simulink model "PR_data"  (R2024a)
settings: Solver=ode45  StartTime=0.0  StopTime=stoptime  RelTol=1e-3
values from neighbouring files (symbols this model uses):
  amp_factor = [0.15; 0.03]/pi*180    [robotparam.m]
  I_est = 1e-3    (= 0.001)    [robotparam.m]
  ifreslosetrack = false    [robotparam.m]    (also in run_data_kick.m; run_data_losetrack.m = true; run_data_noise.m)
  ifresnoise = false    [robotparam.m]    (also in run_data_kick.m; run_data_losetrack.m; run_data_noise.m = true)
  ifrobotkicking = false    [robotparam.m]    (also in run_data_kick.m = true; run_data_losetrack.m; run_data_noise.m; run_sim.m = true)
  ifrobotnoise = false    [robotparam.m]    (also in run_data_kick.m; run_data_losetrack.m; run_data_noise.m = true)
  motor1mid = 0.445*180    (= 80.1)    [robotparam.m]    (also in run_receive.m)
  motor2mid = 0.45*180    (= 81)    [robotparam.m]    (also in run_receive.m)
  ref_theta = 0    [robotparam.m]    (also in run_data_kick.m = 3.14159265359; run_data_losetrack.m = 3.14159265359; run_data_noise.m = 3.14159265359; run_sim.m = 3.14159265359)
  ref_thetadot = 0    [robotparam.m]    (also in run_data_kick.m; run_data_losetrack.m; run_data_noise.m; run_sim.m)
  res_losetrack_period = 5    [robotparam.m]    (also in run_data_kick.m; run_data_losetrack.m = list(i,2); run_data_noise.m)
  res_losetrack_start = 9    [robotparam.m]    (also in run_data_kick.m; run_data_losetrack.m = list(i,1); run_data_noise.m)
  res_noise_seed = round(10000*[rand() rand()])    [robotparam.m]    (also in run_data_kick.m; run_data_losetrack.m; run_data_noise.m = [list(i,4) list(i,5)])
  res_noise_variance = 0.01*[1 1]    [robotparam.m]    (also in run_data_kick.m; run_data_losetrack.m; run_data_noise.m = [list(i,3) list(i,3)])
  robot_kick_height = 0    [robotparam.m]    (also in run_data_kick.m; run_data_losetrack.m; run_data_noise.m; run_sim.m = 1)
  robot_kick_period = 0.1    [robotparam.m]    (also in run_data_kick.m; run_data_losetrack.m; run_data_noise.m; run_sim.m)
  robot_kick_start = 10    [robotparam.m]    (also in run_data_kick.m = 30; run_data_losetrack.m; run_data_noise.m; run_sim.m = 1020)
  robot_noise_seed = round(10000*rand())    [robotparam.m]    (also in run_data_kick.m; run_data_losetrack.m; run_data_noise.m = list(i,2))
  robot_noise_variance = 0.0001    [robotparam.m]    (also in run_data_kick.m; run_data_losetrack.m; run_data_noise.m = list(i,1))
  robot_pendepth = 0.02    [robotparam.m]
  robot_penlength = 0.20    (= 0.2)    [robotparam.m]
  robot_penwidth = 0.02    [robotparam.m]
  robot_pulse_freq = 0.05    [robotparam.m]    (also in run_data_kick.m = list(i,1); run_data_losetrack.m = 0.5; run_data_noise.m = 0.5; run_sim.m = 0.01)
  robot_pulse_hight = 0.5    [robotparam.m]    (also in run_data_kick.m = list(i,2); run_data_losetrack.m; run_data_noise.m; run_sim.m = 0.08)
  robot_pulse_period = 0.1*100    (= 10)    [robotparam.m]    (also in run_data_kick.m; run_data_losetrack.m; run_data_noise.m; run_sim.m)
  robot_pulse_start = 60    [robotparam.m]    (also in run_data_kick.m = 30; run_data_losetrack.m = 10; run_data_noise.m = 10; run_sim.m = 1020)
  robot_sphere_mass = 0.1    [robotparam.m]
  s = {s1, s2}    [run_receive.m]
  samplingrate = 0.01    [robotparam.m]
  torquelim = 0.25*robot_penrho*robot_penlength*robot_penwidth*robot_pendepth*robot_penlength/2*g    (= 0.0196133)    [robotparam.m]
  Wout = 0*ones(3,1+4+2)    [robotparam.m]    (also in trainres.m = Woutmat)
  X = SS([1:3 6:end],:)    [trainres.m]
  Y = tar{i}    [trainres.m]
undefined symbols (not defined in the file or in its folder): arm_radius, arm_radius_previus, spring_position_scale, Z
libraries: sm_lib x9, nesl_utility x6, slrealtimeiplib x4, simulink x2, sldrtlib x1, slrealtimeutilitieslib x1, dspindex x1
settings Model: Creator=dante  LastModifiedBy=dante
settings SolverCC: AutoInsertRateTranBlk=on
settings OptimizationCC: DefaultParameterBehavior=Inlined  EnhancedBackFolding=on  PassReuseOutputArgsAs=Individual arguments  ZeroExternalMemoryAtStartup=off  ZeroInternalMemoryAtStartup=off  MaxStackSize=64  OptimizeBlockOrder=speed  DifferentSizesBufferReuse=on  OptimizationCustomize=off  EfficientTunableParamExpr=on
settings DebuggingCC: AlgebraicLoopMsg=none  ParameterTunabilityLossMsg=error
settings HardwareCC: ProdBitPerInt=16  ProdBitPerPointer=16  ProdBitPerSizeT=16  ProdBitPerPtrDiffT=16  ProdLargestAtomicFloat=None  ProdWordSize=8  ProdHWDeviceType=Atmel->AVR
settings SFSimCC: MATLABDynamicMemAlloc=off
settings RTWCC: Description=Embedded Coder  SystemTargetFile=ert.tlc  TemplateMakefile=ert_default_tmf  Toolchain=Arduino AVR  BuildConfiguration=Faster Runs
settings CodeAppCC: ForceParamTrailComments=on  IgnoreCustomStorageClasses=off  OperatorAnnotations=on  SimulinkDataObjDesc=on  SFDataObjDesc=on  InsertBlockDesc=on
settings ERTTargetCC: SupportContinuousTime=on  ExtModeTransport=3  ExtModeStaticAlloc=on  ExtModeStaticAllocSize=250  ExtModeMexFile=ext_xcp  ExtModeIntrfLevel=Level2 - Open  ERTCustomFileTemplate=example_file_process.tlc
settings ExplorerConfigSet: InternalSimMechanicsExplorerSettings="<ExplorerConfiguration><canonicalview>default</canonicalview><AnimationSetting><BasePlaybackSpeed>1.0</BasePlaybackSpeed><PlaybackSpeedFactor>1.0</PlaybackSpeedFactor></AnimationSetting><TilePanel><TileInfo><Tiles Columns=\"1\" Count=\"1\" Rows=\"1\"><Column Weight=\"1\"/><Row Weight=\"1\"/><Tile Height=\"1\" Width=\"1\" X=\"0\" Y=\"0\"/></Tiles></TileInfo><SceneInfo><SceneViewer><BGColor><R>1</R><G>1</G><B>1</B></BGColor><Camera><DoPerspective>off</DoPerspective><Position><X>-6.72546141640504441e-05</X><Y>-1.00004999683291818</Y><Z>0.290146129229805205</Z></Position><Center><X>-6.72546141640504441e-05</X><Y>-4.99968329182032267e-05</Y><Z>0.290146129229805205</Z></Center><Up><X>0</X><Y>-0</Y><Z>1</Z></Up><ViewLimDist>1</ViewLimDist><YLim>0.252627686260521567</YLim><XLim>0.252627686260521567</XLim></Camera></SceneViewer></SceneInfo></TilePanel><MechEditorPanel><Cameras/><GfxPanelCameraMap/><VideoCreator><PlaybackSpeedRatio>1.0</PlaybackSpeedRatio><FrameRate>30</FrameRate><VideoFormat>Motion JPEG AVI</VideoFormat><FrameSize>auto</FrameSize></VideoCreator></MechEditorPanel></ExplorerConfiguration>"

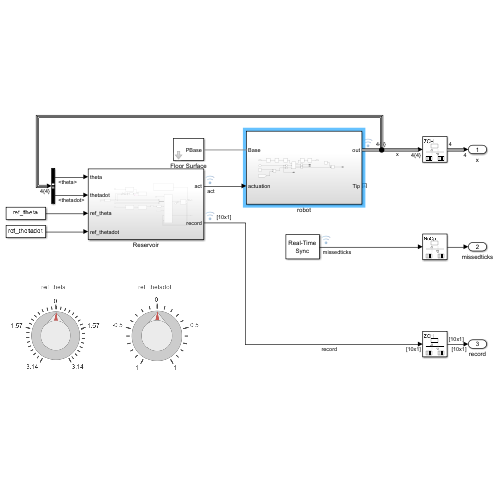
[thumbnail: Simulink's stored preview of the top-level diagram]
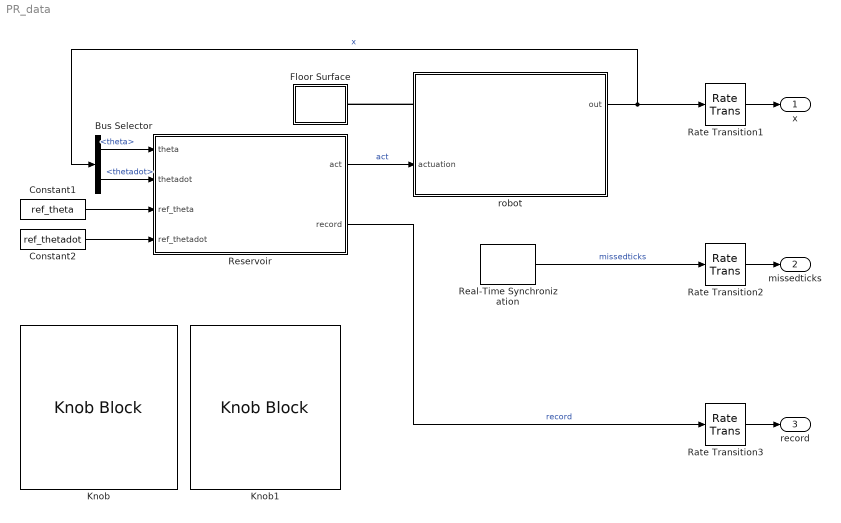
== system PR_data ==
  Bus Selector : BusSelector  OutputSignals=theta,thetadot
  Constant1 : Constant  Value=ref_theta
  Constant2 : Constant  Value=ref_thetadot
  Floor Surface : Subsystem  mask{length=0.5, width=0.5}
      mask prompts: length "grid length [m]"; width "grid width [m]"
  Knob : KnobBlock  ScaleMin=-3.14  ScaleMax=3.14  TickInterval=1.57
  Knob1 : KnobBlock  ScaleMin=-1  ScaleMax=1  TickInterval=0.5
  Rate Transition1 : RateTransition  OutPortSampleTime=samplingrate
  Rate Transition2 : RateTransition  OutPortSampleTime=samplingrate
  Rate Transition3 : RateTransition  OutPortSampleTime=samplingrate
  Real-Time Synchronization : sldrtlib/Real-Time Synchronization  SampleTime=samplingrate  MaxMissedTicks=1000  ShowMissedTicks=on  YieldWhenWaiting=off
  Reservoir : Subsystem
  robot : Subsystem
      settings: PortSchema="{\"entries\":[{\"content\":{\"sides\":[{\"content\":{\"connectorIds\":[\"LConn1\",\"In1\"]},\"type\":\"ConnectorPlacement.EquallySpacedRectSide\",\"uuid\":\"dab85734-5223-47c8-98b4-c5bd2646397a\"},{\"content\":{\"connectorIds\":[\"Out1\",\"RConn1\"],\"side\":\"RIGHT\"},\"type\":\"ConnectorPlacement.EquallySpacedRectSide\",\"uuid\":\"c0ea15e2-5ad4-47fa-8aeb-0218d5c494db\"},{\"content\":{\"side\":\"TOP\"},\"type\":\"ConnectorPlacement.EquallySpacedRectSide\",\"uuid\":\"166100d5-86a1-4512-901d-80935eea9023\"}]},\"type\":\"ConnectorPlacement.EquallySpacedConnector\",\"uuid\":\"1b956e2c-5409-4c92-995b-8a7c87877ed0\"}],\"packageUris\":[\"http://schema.mathworks.com/mf0/Connector/R2020b\"],\"version\":\"1.0\"}"
  x : Outport
  missedticks : Outport  Port=2
  record : Outport  Port=3
  wires:
  robot/1(out) -> Bus Selector/1, Rate Transition1/1  "x"
  Real-Time Synchronization/1 -> Rate Transition2/1  "missedticks"
  Constant2/1 -> Reservoir/4(ref_thetadot)
  Constant1/1 -> Reservoir/3(ref_theta)
  Reservoir/2(record) -> Rate Transition3/1  "record"
  Rate Transition1/1 -> x/1
  Rate Transition2/1 -> missedticks/1
  Rate Transition3/1 -> record/1
  Bus Selector/1 -> Reservoir/1(theta)  "<theta>"
  Bus Selector/2 -> Reservoir/2(thetadot)  "<thetadot>"
  Reservoir/1(act) -> robot/1(actuation)  "act"
  connections:
  robot/LConn1 -- Floor Surface/RConn1

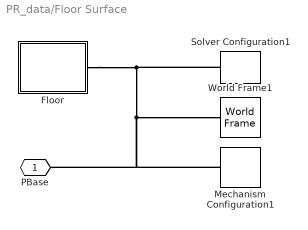
== system PR_data/Floor Surface ==
  Floor : Subsystem
  Mechanism Configuration1 : sm_lib/Utilities/Mechanism Configuration  UniformGravity=Constant  GravityVector=[0 0 -9.80665]  GravityVectorUnits=m/s^2  LinearizationDelta=0.001  JointModeTransitionNonlinearIterations=2
  Solver Configuration1 : nesl_utility/Solver Configuration  PhysicalDomain=network_engine_domain  SubClassName=solver  LeftPortType=input  RightPortType=generic  Tones=[]  Harmonics=[]  SimulateNoise=off  Profile=off  UseLocalSampling=off  EnableSwitchedLinearOptims=on  FrequencyDomain=off  UseCCode=off  RelTol=0.001  AbsTol=1e-06  MinStep=1e-09  ToWorkspace=off  RevertToSquareIcSolve=off  NumHomotopyIterations=100  PhasorMode=off  PhasorModeNumHarmonics=1  ConsistencySolver=NEWTON_FTOL  IndexReductionMethod=DerivativeReplacement  DoDC=off  ResidualTolerance=1e-09  ConsistencyTolSource=GLOBAL  ConsistencyAbsTol=0.001  ConsistencyRelTol=0.001  ConsistencyTolFactor=0.001  UseLocalSolver=off  LocalSolverChoice=NE_BACKWARD_EULER_ADVANCER  ResolveIndetEquations=on  FunctionEvalNumThread=1  LocalSolverSampleTime=0.0002  DoFixedCost=off  MaxNonlinIter=10  MaxModeIter=2  ComputeImpulses=off  ImpulseIterations=2  LinearAlgebra=Sparse  LinearAlgebraNumThread=0  EquationFormulation=NE_TIME_EF  DelaysMemoryBudget=1024  AutomaticFiltering=off  FilteringTimeConstant=0.001  PartitionStorageMethod=AS_NEEDED  PartitionMemoryBudget=1024  PartitionMethod=FAST  MultibodyUseLocalSolver=off  MultibodyLocalSolverChoice=ODE1  MultibodyLocalSolverSampleTime=0.001
  World Frame1 : sm_lib/Frames and Transforms/World Frame
  PBase : PMIOPort  Side=Right
  connections:
  Floor/RConn1 -- PBase/RConn1 -- Mechanism Configuration1/RConn1 -- World Frame1/RConn1 -- Solver Configuration1/RConn1

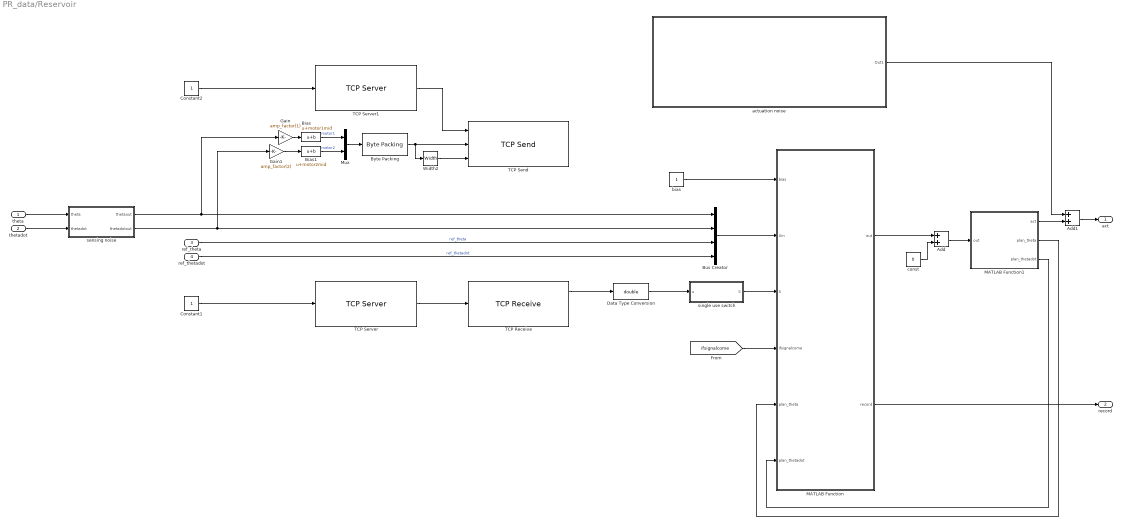
== system PR_data/Reservoir ==
  theta : Inport
  thetadot : Inport  Port=2
  ref_theta : Inport  Port=3
  ref_thetadot : Inport  Port=4
  Add : Sum
  Add1 : Sum
  Bias : Bias  Bias=motor1mid  SaturateOnIntegerOverflow=off
  Bias1 : Bias  Bias=motor2mid  SaturateOnIntegerOverflow=off
  Bus Creator : BusCreator  Inputs=4
  "Byte Packing " : slrealtimeutilitieslib/Byte Packing  MaskPackedDataType=uint8  MaskUnpackedDataTypes={'double'}  MaskAlignment=1
  Constant1 : Constant
  Constant2 : Constant
  Data Type Conversion : DataTypeConversion  OutDataTypeStr=double  SaturateOnIntegerOverflow=off  RndMeth=Floor
  Gain : Gain  Gain=amp_factor(1)
  Gain1 : Gain  Gain=amp_factor(2)
  MATLAB Function : MATLAB Function  TreatAsAtomicUnit=on
  MATLAB Function1 : MATLAB Function  TreatAsAtomicUnit=on
  Mux : Mux  Inputs=2
  TCP Receive : slrealtimeiplib/TCP Receive  socketAddPortVal=Server: 169.254.170.51:65432  rcvWidth=2  sampleTime=-1
  TCP Send : slrealtimeiplib/TCP Send  socketAddPortVal=Server: 169.254.170.51:65431  sampleTime=-1
  TCP Server : slrealtimeiplib/TCP Server  Priority=-1  useHostTargetConn=off  serverAddress=169.254.170.51  serverPort=65432
  TCP Server1 : slrealtimeiplib/TCP Server  Priority=-1  useHostTargetConn=off  serverAddress=169.254.170.51  serverPort=65431
  Width2 : Width
  actuation noise : Subsystem
  bias : Constant
  const : Constant  Value=0
  sensing noise : Subsystem
  single use switch : Subsystem
  act : Outport
  record : Outport  Port=2
  wires:
  TCP Server/1 -> TCP Receive/1
  Constant1/1 -> TCP Server/1
  ref_thetadot/1 -> Bus Creator/4  "ref_thetadot"
  ref_theta/1 -> Bus Creator/3  "ref_theta"
  Bus Creator/1 -> MATLAB Function/2(Xin)
  TCP Receive/1 -> Data Type Conversion/1
  bias/1 -> MATLAB Function/1(bias)
  MATLAB Function/1(out) -> Add/1
  const/1 -> Add/2
  Add/1 -> MATLAB Function1/1(out)
  MATLAB Function/2(record) -> record/1
  Mux/1 -> "Byte Packing "/1
  Width2/1 -> TCP Send/3
  "Byte Packing "/1 -> Width2/1, TCP Send/2
  Gain/1 -> Bias/1
  Gain1/1 -> Bias1/1
  Bias1/1 -> Mux/2  "motor2"
  Bias/1 -> Mux/1  "motor1"
  Constant2/1 -> TCP Server1/1
  TCP Server1/1 -> TCP Send/1
  Data Type Conversion/1 -> single use switch/1(u)
  single use switch/1(S) -> MATLAB Function/3(S)
  MATLAB Function1/2(plan_theta) -> MATLAB Function/5(plan_theta)
  MATLAB Function1/3(plan_thetadot) -> MATLAB Function/6(plan_thetadot)
  [ifsignalcome] -> MATLAB Function/4(ifsignalcome)
  MATLAB Function1/1(act) -> Add1/2
  Add1/1 -> act/1
  actuation noise/1(Out1) -> Add1/1
  sensing noise/1(thetaout) -> Bus Creator/1, Gain/1
  sensing noise/2(thetadotout) -> Bus Creator/2, Gain1/1
  theta/1 -> sensing noise/1(theta)
  thetadot/1 -> sensing noise/2(thetadot)

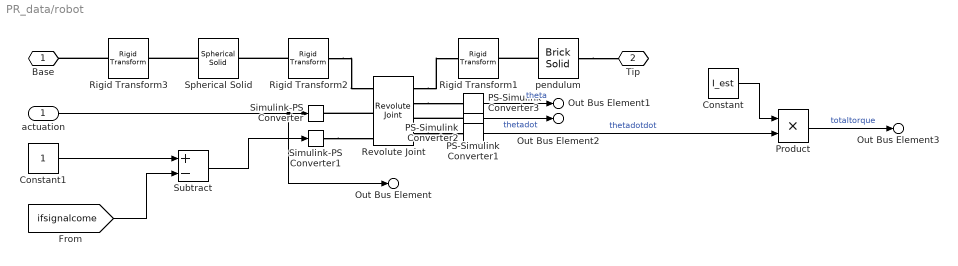
== system PR_data/robot ==
  actuation : Inport
  Constant : Constant  Value=I_est
  Constant1 : Constant
  PS-Simulink Converter1 : nesl_utility/PS-Simulink Converter  PhysicalDomain=network_engine_domain  SubClassName=ps_output  LeftPortType=input  RightPortType=output  PseudoPeriodic=off  Frequencies=[]  VectorFormat=1-D array  Unit=1  AffineConversion=off
  PS-Simulink Converter2 : nesl_utility/PS-Simulink Converter  PhysicalDomain=network_engine_domain  SubClassName=ps_output  LeftPortType=input  RightPortType=output  PseudoPeriodic=off  Frequencies=[]  VectorFormat=1-D array  Unit=1  AffineConversion=off
  PS-Simulink Converter3 : nesl_utility/PS-Simulink Converter  PhysicalDomain=network_engine_domain  SubClassName=ps_output  LeftPortType=input  RightPortType=output  PseudoPeriodic=off  Frequencies=[]  VectorFormat=1-D array  Unit=1  AffineConversion=off
  Product : Product
  Revolute Joint : sm_lib/Joints/Revolute Joint  JointMode=ProvidedByInput  CompositeWrenchDir=FollowerOnBase  CompositeWrenchFrame=BaseFrame  SenseConstraintForce=off  SenseConstraintTorque=off  SenseTotalForce=off  SenseTotalTorque=off  PositionTargetSpecify=on  PositionTargetPriority=Low  PositionTargetValue=robot_ini_theta_p  PositionTargetValueUnits=rad  VelocityTargetSpecify=on  VelocityTargetPriority=Low  VelocityTargetValue=robot_ini_thetadot_p  VelocityTargetValueUnits=rad/s  EquilibriumPosition=0  EquilibriumPositionUnits=rad  SpringStiffness=0  SpringStiffnessUnits=N*m/rad  DampingCoefficient=robot_damping_coeff  DampingCoefficientUnits=N*m/(rad/s)  LowerLimitSpecify=off  LowerLimitBound=-90  LowerLimitBoundUnits=deg  LowerLimitStiffness=1e4  LowerLimitStiffnessUnits=N*m/deg  LowerLimitDamping=10  LowerLimitDampingUnits=N*m/(deg/s)  LowerLimitTransitionRegionWidth=0.1  LowerLimitTransitionRegionWidthUnits=deg  UpperLimitSpecify=off  UpperLimitBound=90  UpperLimitBoundUnits=deg  UpperLimitStiffness=1e4  UpperLimitStiffnessUnits=N*m/deg  UpperLimitDamping=10  UpperLimitDampingUnits=N*m/(deg/s)  UpperLimitTransitionRegionWidth=0.1  UpperLimitTransitionRegionWidthUnits=deg  TorqueActuationMode=InputTorque  MotionActuationMode=ComputedMotion  SensePosition=on  SenseVelocity=on  SenseAcceleration=on  SenseTorqueForce=off  SenseLowerLimitTorqueForce=off  SenseUpperLimitTorqueForce=off
  Rigid Transform1 : sm_lib/Frames and Transforms/Rigid Transform  RotationMethod=AlignedAxes  FollAlignAxisA=+X  BaseAlignAxisA=+X  FollAlignAxisB=-Z  BaseAlignAxisB=+Y  RotationStandardAxis=+Z  RotationAngle=180  RotationAngleUnits=deg  RotationArbitraryAxis=[0 0 1]  RotationSequenceAxes=FollowerAxes  RotationSequence=XYX  RotationSequenceAngles=[0 0 0]  RotationSequenceAnglesUnits=deg  RotationMatrix=[1 0 0; 0 1 0; 0 0 1]  Quaternion=[1 0 0 0]  TranslationMethod=None  TranslationCartesianOffset=[arm_radius*spring_position_scale 0 0]  TranslationCartesianOffsetUnits=m  TranslationStandardAxis=+Z  TranslationStandardOffset=0  TranslationStandardOffsetUnits=m  TranslationROffset=arm_radius_previus*spring_position_scale  TranslationROffsetUnits=m  TranslationThetaOffset=theta  TranslationThetaOffsetUnits=deg  TranslationZOffset=0  TranslationZOffsetUnits=m
  Rigid Transform2 : sm_lib/Frames and Transforms/Rigid Transform  RotationMethod=AlignedAxes  FollAlignAxisA=+X  BaseAlignAxisA=+X  FollAlignAxisB=+Y  BaseAlignAxisB=+Z  RotationStandardAxis=+Z  RotationAngle=180  RotationAngleUnits=deg  RotationArbitraryAxis=[0 0 1]  RotationSequenceAxes=FollowerAxes  RotationSequence=XYX  RotationSequenceAngles=[0 0 0]  RotationSequenceAnglesUnits=deg  RotationMatrix=[1 0 0; 0 1 0; 0 0 1]  Quaternion=[1 0 0 0]  TranslationMethod=None  TranslationCartesianOffset=[arm_radius*spring_position_scale 0 0]  TranslationCartesianOffsetUnits=m  TranslationStandardAxis=+Z  TranslationStandardOffset=0  TranslationStandardOffsetUnits=m  TranslationROffset=arm_radius_previus*spring_position_scale  TranslationROffsetUnits=m  TranslationThetaOffset=theta  TranslationThetaOffsetUnits=deg  TranslationZOffset=0  TranslationZOffsetUnits=m
  Rigid Transform3 : sm_lib/Frames and Transforms/Rigid Transform  RotationMethod=None  FollAlignAxisA=+X  BaseAlignAxisA=+X  FollAlignAxisB=+Y  BaseAlignAxisB=+Z  RotationStandardAxis=+Z  RotationAngle=180  RotationAngleUnits=deg  RotationArbitraryAxis=[0 0 1]  RotationSequenceAxes=FollowerAxes  RotationSequence=XYX  RotationSequenceAngles=[0 0 0]  RotationSequenceAnglesUnits=deg  RotationMatrix=[1 0 0; 0 1 0; 0 0 1]  Quaternion=[1 0 0 0]  TranslationMethod=StandardAxis  TranslationCartesianOffset=[arm_radius*spring_position_scale 0 0]  TranslationCartesianOffsetUnits=m  TranslationStandardAxis=+Z  TranslationStandardOffset=robot_penposz  TranslationStandardOffsetUnits=m  TranslationROffset=arm_radius_previus*spring_position_scale  TranslationROffsetUnits=m  TranslationThetaOffset=theta  TranslationThetaOffsetUnits=deg  TranslationZOffset=0  TranslationZOffsetUnits=m
  Simulink-PS Converter : nesl_utility/Simulink-PS Converter  PhysicalDomain=network_engine_domain  SubClassName=ps_input  LeftPortType=input  RightPortType=output  PseudoPeriodic=off  Frequencies=[]  NoiseDistribution=none  NoiseParameters=[]  Unit=1  AffineConversion=off  FilteringAndDerivatives=provide  SimscapeFilterOrder=1  InputFilterTimeConstant=0.001  UdotUserProvided=0
  Simulink-PS Converter1 : nesl_utility/Simulink-PS Converter  PhysicalDomain=network_engine_domain  SubClassName=ps_input  LeftPortType=input  RightPortType=output  PseudoPeriodic=off  Frequencies=[]  NoiseDistribution=none  NoiseParameters=[]  Unit=1  AffineConversion=off  FilteringAndDerivatives=zero  SimscapeFilterOrder=1  InputFilterTimeConstant=0.001  UdotUserProvided=0
  Spherical Solid : sm_lib/Body Elements/Spherical Solid  SphereRadius=robot_sphere_radius  SphereRadiusUnits=m  ExportEntireGeometry=off  InertiaType=CalculateFromGeometry  BasedOnType=Mass  Density=1000  DensityUnits=kg/m^3  Mass=robot_sphere_mass  MassUnits=kg  CenterOfMass=[0 0 0]  CenterOfMassUnits=m  MomentsOfInertia=[1 1 1]  MomentsOfInertiaUnits=kg*m^2  ProductsOfInertia=[0 0 0]  ProductsOfInertiaUnits=kg*m^2  GraphicType=FromGeometry  MarkerShape=Sphere  MarkerSize=10  GraphicVisPropType=SimpleVisualProperties  GraphicDiffuseColor=[0.8 0.8 0.8]  GraphicOpacity=1.0  GraphicSpecularColor=[0.5 0.5 0.5 1.0]  GraphicAmbientColor=[0.15 0.15 0.15 1.0]  GraphicEmissiveColor=[0.0 0.0 0.0 1.0]  GraphicShininess=75  DoExposeReferenceFrame=on  SerializedFrames=<Frames><Frame><Id>Frame1</Id><Value><Name>F1</Name><Origin><Source>ReferenceFrame</Source><FeatureName></FeatureName></Origin><PrimaryAxis><DefinedDirection>+Z</DefinedDirection><Source>ReferenceFrame</Source><SourceDirection>+Z</SourceDirection><FeatureName></FeatureName></PrimaryAxis><SecondaryAxis><DefinedDirection>+X</DefinedDirection><Source>ReferenceFrame</Source><SourceDirection>+X</SourceDirection><FeatureName></FeatureName></SecondaryAxis></Value></Frame></Frames>
  Subtract : Sum  Inputs=+-
  pendulum : sm_lib/Body Elements/Brick Solid  BrickDimensions=[robot_penwidth robot_pendepth robot_penlength]  BrickDimensionsUnits=m  ExportEntireGeometry=off  InertiaType=CalculateFromGeometry  BasedOnType=Density  Density=robot_penrho  DensityUnits=kg/m^3  Mass=1  MassUnits=kg  CenterOfMass=[0 0 0]  CenterOfMassUnits=m  MomentsOfInertia=[1 1 1]  MomentsOfInertiaUnits=kg*m^2  ProductsOfInertia=[0 0 0]  ProductsOfInertiaUnits=kg*m^2  GraphicType=FromGeometry  MarkerShape=Sphere  MarkerSize=10  GraphicVisPropType=SimpleVisualProperties  GraphicDiffuseColor=[0.0 0.4 1.0]  GraphicOpacity=1.0  GraphicSpecularColor=[0.5 0.5 0.5 1.0]  GraphicAmbientColor=[0.15 0.15 0.15 1.0]  GraphicEmissiveColor=[0.0 0.0 0.0 1.0]  GraphicShininess=75  DoExposeReferenceFrame=off  SerializedFrames=<Frames><Frame><Id>Frame1</Id><Value><Name>F1</Name><Origin><Source>GeometricFeature</Source><FeatureName>-z surface</FeatureName></Origin><PrimaryAxis><DefinedDirection>+Z</DefinedDirection><Source>ReferenceFrame</Source><SourceDirection>+Z</SourceDirection><FeatureName></FeatureName></PrimaryAxis><SecondaryAxis><DefinedDirection>+X</DefinedDirection><Source>ReferenceFrame</Source><SourceDirection>+X</SourceDirection><FeatureName></FeatureName></SecondaryAxis></Value></Frame><Frame><Id>Frame2</Id><Value><Name>F2</Name><Origin><Source>GeometricFeature</Source><FeatureName>+z surface</FeatureName></Origin><PrimaryAxis><DefinedDirection>+Z</DefinedDirection><Source>ReferenceFrame</Source><SourceDirection>-Z</SourceDirection><FeatureName></FeatureName></PrimaryAxis><SecondaryAxis><DefinedDirection>+X</DefinedDirection><Source>ReferenceFrame</Source><SourceDirection>+X</SourceDirection><FeatureName></FeatureName></SecondaryAxis></Value></Frame></Frames>
  Base : PMIOPort  Side=Left
  Tip : PMIOPort  Port=2  Side=Right
  Out Bus Element1 : Outport  PortName=out  Element=theta
  Out Bus Element2 : Outport  PortName=out  Element=thetadot
  Out Bus Element3 : Outport  PortName=out  Element=totaltorque
  Out Bus Element : Outport  PortName=out  Element=actuationtorque
  wires:
  PS-Simulink Converter3/1 -> Out Bus Element1/1  "theta"
  PS-Simulink Converter1/1 -> Out Bus Element2/1  "thetadot"
  PS-Simulink Converter2/1 -> Product/2  "thetadotdot"
  Product/1 -> Out Bus Element3/1  "totaltorque"
  Constant/1 -> Product/1
  actuation/1 -> Simulink-PS Converter/1, Out Bus Element/1
  Subtract/1 -> Simulink-PS Converter1/1
  Constant1/1 -> Subtract/1
  [ifsignalcome] -> Subtract/2
  connections:
  Revolute Joint/LConn2 -- Simulink-PS Converter/RConn1
  Revolute Joint/RConn2 -- PS-Simulink Converter3/LConn1
  Rigid Transform2/LConn1 -- Spherical Solid/RConn1
  PS-Simulink Converter1/LConn1 -- Revolute Joint/RConn3
  Spherical Solid/LConn1 -- Rigid Transform3/RConn1
  pendulum/LConn1 -- Rigid Transform1/RConn1
  Rigid Transform3/LConn1 -- Base/RConn1
  pendulum/RConn1 -- Tip/RConn1
  Rigid Transform2/RConn1 -- Revolute Joint/LConn1
  Revolute Joint/RConn4 -- PS-Simulink Converter2/LConn1
  Revolute Joint/RConn1 -- Rigid Transform1/LConn1
  Simulink-PS Converter1/RConn1 -- Revolute Joint/LConn3

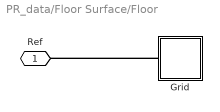
== system PR_data/Floor Surface/Floor ==
  Grid : Subsystem  mask(Grid Lines){grid_origin=[-length -width 0], grid_size=[length width], grid_linewidth=0.001, grid_num_squares=20, grid_color=[0.8 0.8 0.8], grid_opacity=0.8}
      mask prompts: grid_origin "Origin (m)"; grid_size "Arena size (m)"; grid_linewidth "Grid Line Width (m)"; grid_num_squares "Number of Squares"; grid_color "Grid Color [RGB]"; grid_opacity "Grid Opacity (0-1)"
      mask help: Creates grids on 3 planes XZ, YZ, and XZ.
      mask init:
      | mesh_xsec = Extr_Data_Mesh(grid_size(1), grid_size(2), grid_num_squares, grid_num_squares, grid_size(1)/grid_num_squares-grid_linewidth, grid_size(2)/grid_num_squares-grid_linewidth);
  Ref : PMIOPort  Side=Right
  connections:
  Grid/LConn1 -- Ref/RConn1

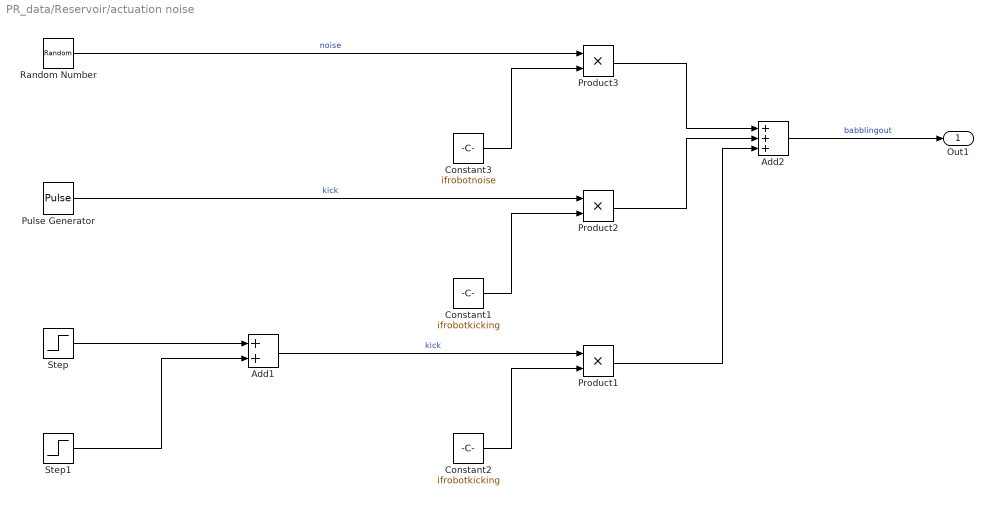
== system PR_data/Reservoir/actuation noise ==
  Add1 : Sum
  Add2 : Sum  Inputs=+++
  Constant1 : Constant  Value=ifrobotkicking
  Constant2 : Constant  Value=ifrobotkicking
  Constant3 : Constant  Value=ifrobotnoise
  Product1 : Product
  Product2 : Product
  Product3 : Product
  Pulse Generator : DiscretePulseGenerator  PulseType=Time based  Amplitude=robot_pulse_hight  Period=1/robot_pulse_freq  PulseWidth=robot_pulse_period*robot_pulse_freq  PhaseDelay=robot_pulse_start
  Random Number : RandomNumber  Variance=robot_noise_variance  Seed=robot_noise_seed  SampleTime=samplingrate
  Step : Step  Time=robot_kick_start  After=robot_kick_height  SampleTime=0
  Step1 : Step  Time=robot_kick_start+robot_kick_period  After=-robot_kick_height  SampleTime=0
  Out1 : Outport
  wires:
  Constant2/1 -> Product1/2
  Random Number/1 -> Product3/1  "noise"
  Product1/1 -> Add2/3
  Step/1 -> Add1/1
  Product2/1 -> Add2/2
  Product3/1 -> Add2/1
  Step1/1 -> Add1/2
  Pulse Generator/1 -> Product2/1  "kick"
  Add2/1 -> Out1/1  "babblingout"
  Constant1/1 -> Product2/2
  Constant3/1 -> Product3/2
  Add1/1 -> Product1/1  "kick"

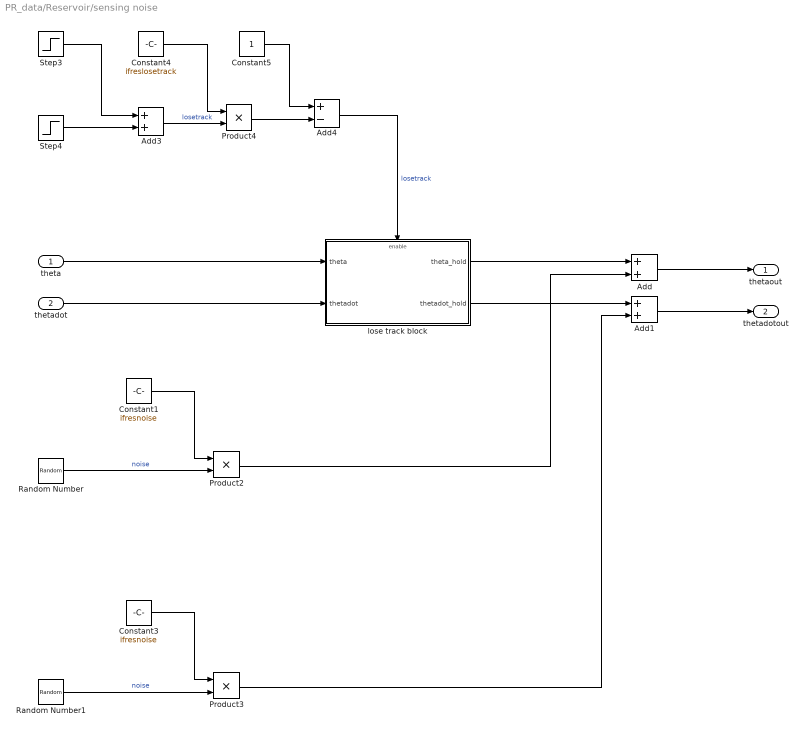
== system PR_data/Reservoir/sensing noise ==
  theta : Inport
  thetadot : Inport  Port=2
  Add : Sum
  Add1 : Sum
  Add3 : Sum
  Add4 : Sum  Inputs=+-
  Constant1 : Constant  Value=ifresnoise
  Constant3 : Constant  Value=ifresnoise
  Constant4 : Constant  Value=ifreslosetrack
  Constant5 : Constant
  Product2 : Product
  Product3 : Product
  Product4 : Product
  Random Number : RandomNumber  Variance=res_noise_variance(1)  Seed=res_noise_seed(1)  SampleTime=samplingrate
  Random Number1 : RandomNumber  Variance=res_noise_variance(2)  Seed=res_noise_seed(2)  SampleTime=samplingrate
  Step3 : Step  Time=res_losetrack_start  SampleTime=0
  Step4 : Step  Time=res_losetrack_start+res_losetrack_period  After=-1  SampleTime=0
  lose track block : Subsystem
  thetaout : Outport
  thetadotout : Outport  Port=2
  wires:
  Step3/1 -> Add3/1
  Add4/1 -> lose track block/Enable  "losetrack"
  Constant5/1 -> Add4/1
  Constant4/1 -> Product4/1
  Step4/1 -> Add3/2
  Product4/1 -> Add4/2
  Add3/1 -> Product4/2  "losetrack"
  thetadot/1 -> lose track block/2(thetadot)
  theta/1 -> lose track block/1(theta)
  Random Number1/1 -> Product3/2  "noise"
  Constant3/1 -> Product3/1
  Product3/1 -> Add1/2
  Constant1/1 -> Product2/1
  Random Number/1 -> Product2/2  "noise"
  Product2/1 -> Add/2
  lose track block/1(theta_hold) -> Add/1
  lose track block/2(thetadot_hold) -> Add1/1
  Add/1 -> thetaout/1
  Add1/1 -> thetadotout/1

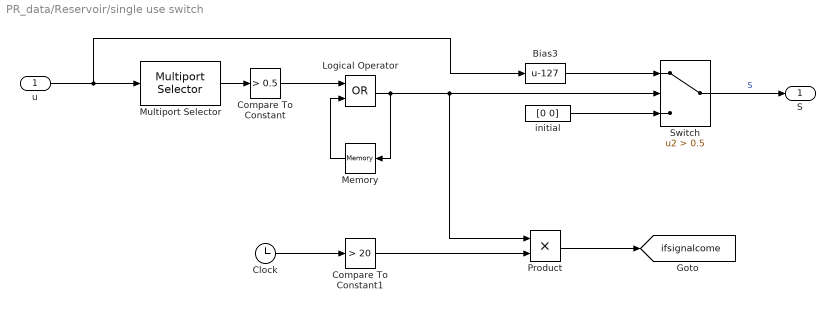
== system PR_data/Reservoir/single use switch ==
  u : Inport
  Bias3 : Bias  Bias=-127  SaturateOnIntegerOverflow=off
  Clock : Clock
  Compare To Constant : simulink/Logic and Bit Operations/Compare To Constant  relop=>  const=0.5  OutDataTypeStr=boolean
  Compare To Constant1 : simulink/Logic and Bit Operations/Compare To Constant  relop=>  const=20  OutDataTypeStr=boolean
  Logical Operator : Logic  Operator=OR  AllPortsSameDT=off  OutDataTypeStr=boolean
  Memory : Memory
  Multiport Selector : dspindex/Multiport Selector  rowsOrCols=Rows  idxCellArray=1  idxErrMode=Clip Index
  Product : Product
  Switch : Switch  Criteria=u2 > Threshold  Threshold=0.5  SaturateOnIntegerOverflow=off  InputSameDT=off
  initial : Constant  Value=[0 0]
  S : Outport
  tag scope: ifsignalcome=global
  wires:
  Switch/1 -> S/1  "S"
  Memory/1 -> Logical Operator/2
  initial/1 -> Switch/3
  Compare To Constant/1 -> Logical Operator/1
  Bias3/1 -> Switch/1
  u/1 -> Multiport Selector/1, Bias3/1
  Logical Operator/1 -> Switch/2, Product/1, Memory/1
  Multiport Selector/1 -> Compare To Constant/1
  Clock/1 -> Compare To Constant1/1
  Compare To Constant1/1 -> Product/2
  Product/1 -> [ifsignalcome]

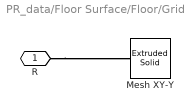
== system PR_data/Floor Surface/Floor/Grid ==
  Mesh XY-Y : sm_lib/Body Elements/Extruded Solid  ExtrusionType=General  PolygonNumSides=3  PolygonOuterRadius=1  PolygonOuterRadiusUnits=m  ExportEntireGeometry=off  ExtrusionCrossSection=mesh_xsec  ExtrusionCrossSectionUnits=m  ExportConvexHullGeometry=off  ExtrusionLength=grid_linewidth  ExtrusionLengthUnits=m  InertiaType=CalculateFromGeometry  BasedOnType=Density  Density=1000  DensityUnits=kg/(m^3)  Mass=1  MassUnits=kg  CenterOfMass=[0 0 0]  CenterOfMassUnits=m  MomentsOfInertia=[1 1 1]  MomentsOfInertiaUnits=kg*m^2  ProductsOfInertia=[0 0 0]  ProductsOfInertiaUnits=kg*m^2  GraphicType=FromGeometry  MarkerShape=Sphere  MarkerSize=10  GraphicVisPropType=SimpleVisualProperties  GraphicDiffuseColor=[0.5 0.5 0.5]  GraphicOpacity=1.0  GraphicSpecularColor=[0.5 0.5 0.5 1.0]  GraphicAmbientColor=[0.15 0.15 0.15 1.0]  GraphicEmissiveColor=[0.0 0.0 0.0 1.0]  GraphicShininess=75  DoExposeReferenceFrame=on  SerializedFrames=<Frames/>
  R : PMIOPort  Side=Left
  connections:
  R/RConn1 -- Mesh XY-Y/RConn1

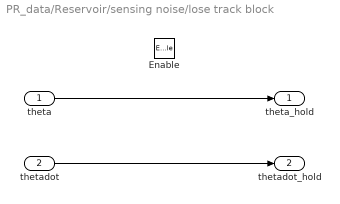
== system PR_data/Reservoir/sensing noise/lose track block ==
  theta : Inport
  thetadot : Inport  Port=2
  Enable : EnablePort
  theta_hold : Outport
  thetadot_hold : Outport  Port=2
  wires:
  theta/1 -> theta_hold/1
  thetadot/1 -> thetadot_hold/1

== matlab function PR_data/Reservoir/MATLAB Function1 ==
  data: out input; act output; plan_theta output; plan_thetadot output
function [act, plan_theta, plan_thetadot] = fcn(out)

    act = out(1,1);
    plan_theta = out(2,1);
    plan_thetadot = out(3,1);

end

== matlab function PR_data/Reservoir/MATLAB Function ==
  data: bias input; out output size=3,1; Xin input size=4; S input; ifsignalcome input; Wout parameter; record output size=10,1; plan_theta input; plan_thetadot input; torquelim parameter
function [out, record] = fcn(bias, Xin, S, ifsignalcome, Wout, plan_theta, plan_thetadot, torquelim)
    S = double(S);

    % XX = [bias; Xin.theta; Xin.thetadot; Xin.plan_theta; Xin.plan_thetadot; Xin.ref_theta; Xin.ref_thetadot; S];
    XX = [bias; Xin(1); Xin(2); plan_theta; plan_thetadot; S];
    out = Wout*XX;

    if out(1) > torquelim
        out(1) = torquelim;
    elseif out(1) < -torquelim
        out(1) = -torquelim;
    end

    n = round((Xin(1) - Xin(3))/(2*pi));

    if abs(Xin(1) - Xin(3) - 2*pi*n) < pi/4
        out(2) = Xin(3) + 2*pi*n;
        out(3) = Xin(4);
    end

    if ~ifsignalcome
        out = [0; 0; 0];
    end

    record = [XX; out];

end
